simulink model "nms3D_2021"  (R2021a)
settings: Solver=ode15s  StartTime=0.0  StopTime=2  MaxStep=1e-2  RelTol=1e-2
StartFcn:
  | tic
StopFcn:
  | toc
  | 
  | 
  | %if GimbalLockFlag
  |  % fprintf(2, 'Almost reached Gimbal Lock of IMU. Simulation stopped.\n')
  | %end
  | 
  | %fprintf('Elapsed time: %4.2f sec (%4.2f%% realtime)\n', a, tout(end)/a*100)
values from neighbouring files (symbols this model uses):
  Balance02 = pMod(24:29)    [AssignSimulinkParams.m]    (also in assign_parameters.m = param(26:29))
  Balance13 = pMod(30:35)    [AssignSimulinkParams.m]    (also in assign_parameters.m = param(30:33))
  BalanceTrunk = pMod(22:23)    [AssignSimulinkParams.m]    (also in assign_parameters.m = param(22:23))
  BalanceTrunkLat = param(24:25)    [assign_parameters.m]
  BalanceTrunkLatOld = pMod(43:46)    [AssignSimulinkParams.m]    (also in assign_parameters.m = param(43:46))
  BalanceTrunkOld = param(49:53)    [assign_parameters.m]
  BasisStim = pMod(1:11)    [AssignSimulinkParams.m]    (also in assign_parameters.m = param(1:11))
  CompliantLeg = pMod(12:14)    [AssignSimulinkParams.m]    (also in assign_parameters.m = param(12:14))
  CompliantLegLat = pMod(15)    [AssignSimulinkParams.m]    (also in assign_parameters.m = param(15))
  PreventKneeOverextension = pMod(16:21)    [AssignSimulinkParams.m]    (also in assign_parameters.m = param(16:21))
  SwingCompLatOld = param(47:48)    [assign_parameters.m]
  Target02 = pMod(36:38)    [AssignSimulinkParams.m]    (also in assign_parameters.m = param(34:36))
  Target02_va = pMod(49:54)    [AssignSimulinkParams.m]    (also in assign_parameters.m = param(60:65))
  Target13 = pMod(39:41)    [AssignSimulinkParams.m]    (also in assign_parameters.m = param(37:39))
  Target13_va = pMod(55:60)    [AssignSimulinkParams.m]    (also in assign_parameters.m = param(66:71))
  theta0_world = param(59)    [assign_parameters.m]
  WramameiSL_1000 = readmatrix('WSL_1000_Norm_Sigmoid_MSE_cont.csv')    [nms3D_prep.m]
  ZramameiSL_1000 = readmatrix('ZSL_1000_Norm_Sigmoid_MSE_cont.csv')    [nms3D_prep.m]
undefined symbols (not defined in the file or in its folder): ICs, mParams, X, Y, Z
libraries: nesl_utility x106, sm_lib x87, simulink x70, eeGeneralControl x28, robotmaniplib x14, dspinverses x10, robotcorelib x5, dspmathops x3, vrlib x1, pid_lib x1
(part 3 of 8)

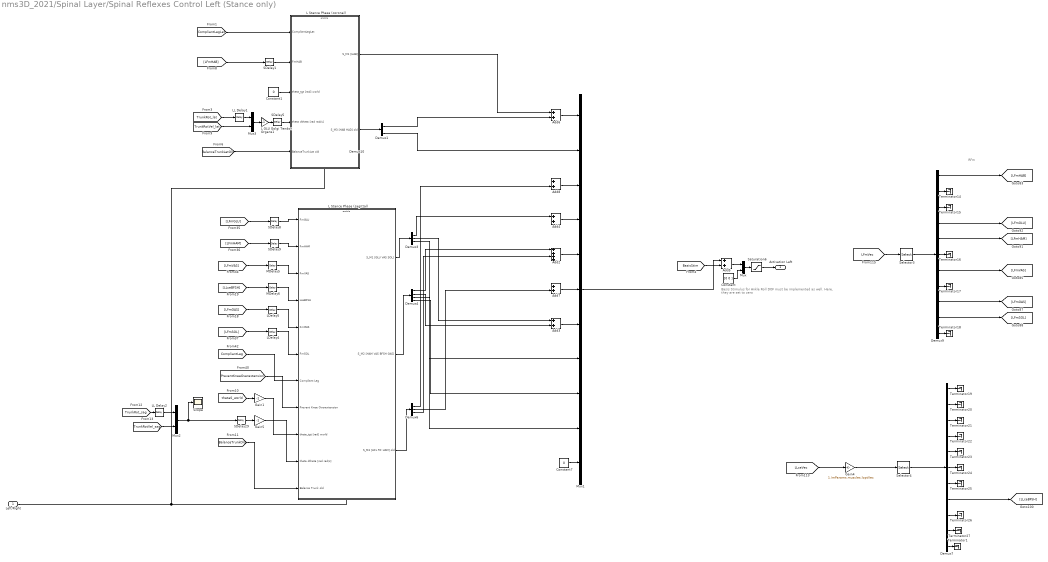
== system nms3D_2021/Spinal Layer/Spinal Reflexes Control Left (Stance only) ==
  note: Basis Stimulus for Ankle Roll DOF must be implemented as well.
      | Here, they are set to zero
  note: RFm
  Left/Right : Inport
  Add2 : Sum  Inputs=++++
  Add{3..8} (6 alike) : Sum
  Constant : Constant  Value=[0 0 ]
  Constant1 : Constant  Value=0
  Constant7 : Constant  Value=0
  Demux1 : Demux  Outputs=2
  Demux10 : Demux  Outputs=2
  Demux3 : Demux  Outputs=3
  Demux4 : Demux
  Demux6 : Demux  Outputs=3
  Demux7 : Demux  Outputs=11
  Demux9 : Demux  Outputs=11
  Gain1 : Gain  Gain=-1
  Gain4 : Gain  Gain=1./mParams.muscles.loptVec
  Gain5 : Gain  Gain=-1
  L GLU Golgi Tendon Organs1 : Gain  Gain=-1
  L Stance Phase (coronal) : Subsystem  TreatAsAtomicUnit=on
  L Stance Phase (sagittal) : Subsystem  TreatAsAtomicUnit=on
  LDelay4 : TransportDelay  DelayTime=mParams.control.delays.long
  LDelay5 : TransportDelay  DelayTime=mParams.control.delays.long
  LL Delay1 : TransportDelay  DelayTime=mParams.control.delays.longloop/2
  LL Delay2 : TransportDelay  DelayTime=mParams.control.delays.longloop/2
  MDelay5 : TransportDelay  DelayTime=mParams.control.delays.mid
  MDelay6 : TransportDelay  DelayTime=mParams.control.delays.mid
  Mux : Mux  Inputs=2
  Mux1 : Mux  Inputs=11
  Mux2 : Mux  Inputs=2
  Mux3 : Mux  Inputs=2
  SDelay{1,5,8..9,29} (5 alike) : TransportDelay  DelayTime=mParams.control.delays.short
  Saturation6 : Saturate  UpperLimit=1  LowerLimit=0.01  ZeroCross=off
  Scope : Scope
  Selector3 : Selector  InputPortWidth=13  IndexOptions=Index vector (dialog)  Indices=[1:11]  OutputSizes=1
  Selector4 : Selector  InputPortWidth=13  IndexOptions=Index vector (dialog)  Indices=[1:11]  OutputSizes=1
  Terminator{1,14..27} (15 alike) : Terminator
  Activation Left : Outport
  wires:
  [LFmVec] -> Selector3/1
  Demux9/1 -> [LFmHAB]
  Gain4/1 -> Selector4/1
  Demux9/5 -> [LFmHAM]
  Demux7/8 -> [LLceBFSH]
  Demux9/9 -> [LFmGAS]
  Demux9/10 -> [LFmSOL]
  Demux9/4 -> [LFmGLU]
  Demux9/7 -> [LFmVAS]
  Demux7/11 -> Terminator1/1
  Saturation6/1 -> Activation Left/1
  Left/Right/1 -> L Stance Phase (sagittal)/Enable, L Stance Phase (coronal)/Enable
  Demux9/2 -> Terminator14/1
  Demux9/3 -> Terminator15/1
  Demux9/6 -> Terminator16/1
  Demux9/8 -> Terminator17/1
  Demux9/11 -> Terminator18/1
  Demux7/1 -> Terminator19/1
  Demux7/2 -> Terminator20/1
  Demux7/3 -> Terminator21/1
  Demux7/4 -> Terminator22/1
  Demux7/5 -> Terminator23/1
  Demux7/6 -> Terminator24/1
  Demux7/7 -> Terminator25/1
  Demux7/9 -> Terminator26/1
  Demux7/10 -> Terminator27/1
  [BasisStim] -> Add5/2
  Mux1/1 -> Add5/1
  Constant7/1 -> Mux1/11
  Add2/1 -> Mux1/5
  Add3/1 -> Mux1/7
  [LFmGLU] -> SDelay8/1
  SDelay9/1 -> L Stance Phase (sagittal)/2(FmHAM)
  MDelay6/1 -> L Stance Phase (sagittal)/4(LceBFSH)
  [LLceBFSH] -> MDelay6/1
  [LFmSOL] -> LDelay4/1
  MDelay5/1 -> L Stance Phase (sagittal)/3(FmVAS)
  [LFmGAS] -> LDelay5/1
  LDelay5/1 -> L Stance Phase (sagittal)/5(FmGAS)
  SDelay8/1 -> L Stance Phase (sagittal)/1(FmGLU)
  [LFmHAM] -> SDelay9/1
  LDelay4/1 -> L Stance Phase (sagittal)/6(FmSOL)
  [LFmVAS] -> MDelay5/1
  [CompliantLeg] -> L Stance Phase (sagittal)/7(Compliant Leg)
  [PreventKneeOverextension] -> L Stance Phase (sagittal)/8(Prevent Knee Overextension)
  [CompliantLegLat] -> L Stance Phase (coronal)/1(CompliantLegLat)
  [LFmHAB] -> SDelay1/1
  Constant1/1 -> L Stance Phase (coronal)/3(theta_tgt [rad] world)
  SDelay1/1 -> L Stance Phase (coronal)/2(FmHAB)
  Add6/1 -> Mux1/1
  SDelay5/1 -> L Stance Phase (coronal)/4(theta dtheta [rad rad/s])
  [TrunkRotVel_lat] -> Mux3/2
  [TrunkRot_lat] -> LL Delay1/1
  LL Delay1/1 -> Mux3/1
  [BalanceTrunkLatOld] -> L Stance Phase (coronal)/5(BalanceTrunkLat old)
  [theta0_world] -> Gain1/1
  Gain1/1 -> L Stance Phase (sagittal)/9(theta_tgt [rad] world)
  Mux2/1 -> Scope/1, SDelay29/1
  SDelay29/1 -> Gain5/1
  LL Delay2/1 -> Mux2/1
  Gain5/1 -> L Stance Phase (sagittal)/10(theta dtheta [rad rad/s])
  [TrunkRot_sag] -> LL Delay2/1
  [TrunkRotVel_sag] -> Mux2/2
  [BalanceTrunkOld] -> L Stance Phase (sagittal)/11(Balance Trunk old)
  Mux3/1 -> L GLU Golgi Tendon Organs1/1
  L GLU Golgi Tendon Organs1/1 -> SDelay5/1
  L Stance Phase (coronal)/1(S_M1 [HAB]) -> Add6/1
  L Stance Phase (coronal)/2(S_M3 [HAB HAD] old) -> Demux1/1
  Demux1/1 -> Add6/2
  Demux1/2 -> Mux1/2
  L Stance Phase (sagittal)/1(S_M1 [GLU VAS SOL]) -> Demux3/1
  L Stance Phase (sagittal)/2(S_M2 [HAM VAS BFSH GAS]) -> Demux4/1
  L Stance Phase (sagittal)/3(S_M3 [HFL RF HAM] old) -> Demux6/1
  Add4/1 -> Mux1/4
  Demux3/1 -> Add4/1
  Demux4/1 -> Add2/1
  Demux6/3 -> Add2/3
  Add7/1 -> Mux1/6
  Add8/1 -> Mux1/3
  Demux6/1 -> Add8/2
  Demux6/2 -> Add7/2
  Demux3/2 -> Add3/1
  Demux4/2 -> Add3/2
  Demux4/3 -> Mux1/8
  Demux4/4 -> Mux1/9
  Demux3/3 -> Mux1/10
  Constant/1 -> Mux/2
  Add5/1 -> Mux/1
  Mux/1 -> Saturation6/1
  Selector3/1 -> Demux9/1
  [LLceVec] -> Gain4/1
  Selector4/1 -> Demux7/1

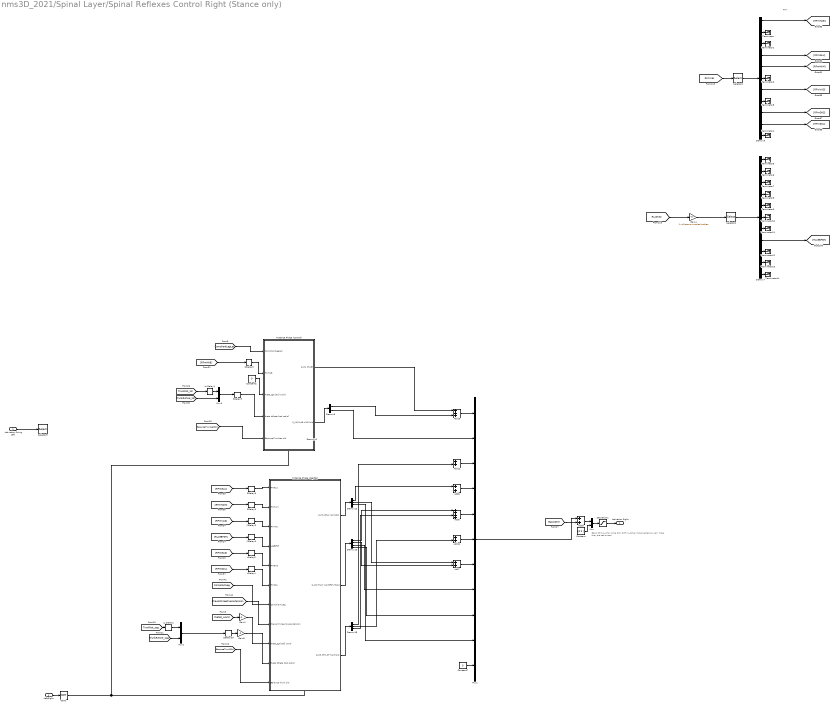
== system nms3D_2021/Spinal Layer/Spinal Reflexes Control Right (Stance only) ==
  note: RFm
  note: Basis Stimulus for Ankle Roll DOF must be implemented as well.
      | Here, they are set to zero
  Left/Right : Inport
  Activation Swing Left : Inport  Port=2
  Add10 : Sum  Inputs=+++
  Add{7..9,11..12} (5 alike) : Sum
  Add6 : Sum  Inputs=++++
  Constant : Constant  Value=[0 0 ]
  Constant1 : Constant  Value=0
  Constant7 : Constant  Value=0
  Demux10 : Demux  Outputs=2
  Demux12 : Demux  Outputs=3
  Demux13 : Demux
  Demux15 : Demux  Outputs=3
  Demux7 : Demux  Outputs=11
  Demux8 : Demux  Outputs=2
  Demux9 : Demux  Outputs=11
  Gain1 : Gain  Gain=-1
  Gain4 : Gain  Gain=1./mParams.muscles.loptVec
  Gain5 : Gain  Gain=-1
  LDelay4 : TransportDelay  DelayTime=mParams.control.delays.long
  LDelay5 : TransportDelay  DelayTime=mParams.control.delays.long
  LL Delay1 : TransportDelay  DelayTime=mParams.control.delays.longloop/2
  LL Delay2 : TransportDelay  DelayTime=mParams.control.delays.longloop/2
  MDelay5 : TransportDelay  DelayTime=mParams.control.delays.mid
  MDelay6 : TransportDelay  DelayTime=mParams.control.delays.mid
  Mux : Mux  Inputs=2
  Mux1 : Mux  Inputs=11
  Mux2 : Mux  Inputs=2
  Mux3 : Mux  Inputs=2
  NOT1 : Logic  Operator=NOT  AllPortsSameDT=off  OutDataTypeStr=boolean
  R Stance Phase (coronal) : Subsystem  TreatAsAtomicUnit=on
  R Stance Phase (sagittal) : Subsystem  TreatAsAtomicUnit=on
  SDelay{3,5,8..9,29} (5 alike) : TransportDelay  DelayTime=mParams.control.delays.short
  Saturation1 : Saturate  UpperLimit=1  LowerLimit=0.01  ZeroCross=off
  Selector1 : Selector  InputPortWidth=13  IndexOptions=Index vector (dialog)  Indices=[1:11]  OutputSizes=1
  Selector2 : Selector  InputPortWidth=13  IndexOptions=Index vector (dialog)  Indices=[1:11]  OutputSizes=1
  Selector5 : Selector  InputPortWidth=13  IndexOptions=Index vector (dialog)  Indices=[1:11]  OutputSizes=1
  Terminator{,1..14} (15 alike) : Terminator
  Activation Right : Outport
  wires:
  [RFmVec] -> Selector1/1
  Demux9/1 -> [RFmHAB]
  Gain4/1 -> Selector2/1
  Demux9/5 -> [RFmHAM]
  Demux7/8 -> [RLceBFSH]
  Demux9/9 -> [RFmGAS]
  Demux9/10 -> [RFmSOL]
  Demux9/4 -> [RFmGLU]
  Demux9/7 -> [RFmVAS]
  Demux7/11 -> Terminator14/1
  Demux9/2 -> Terminator/1
  Demux9/3 -> Terminator1/1
  Demux9/6 -> Terminator2/1
  Demux9/8 -> Terminator3/1
  Demux9/11 -> Terminator4/1
  Demux7/1 -> Terminator5/1
  Demux7/2 -> Terminator6/1
  Demux7/3 -> Terminator7/1
  Demux7/4 -> Terminator8/1
  Demux7/5 -> Terminator9/1
  Demux7/6 -> Terminator10/1
  Demux7/7 -> Terminator11/1
  Demux7/9 -> Terminator12/1
  Demux7/10 -> Terminator13/1
  [RFmHAB] -> SDelay3/1
  LL Delay1/1 -> Mux3/1
  [CompliantLeg] -> R Stance Phase (sagittal)/7(Compliant Leg)
  [theta0_world] -> Gain1/1
  Demux13/1 -> Add6/1
  Left/Right/1 -> NOT1/1
  Gain1/1 -> R Stance Phase (sagittal)/9(theta_tgt [rad] world)
  Demux12/2 -> Add7/1
  [RFmGLU] -> SDelay8/1
  SDelay8/1 -> R Stance Phase (sagittal)/1(FmGLU)
  [RLceBFSH] -> MDelay6/1
  Add6/1 -> Mux1/5
  Demux12/3 -> Mux1/10
  MDelay6/1 -> R Stance Phase (sagittal)/4(LceBFSH)
  Mux3/1 -> SDelay5/1
  R Stance Phase (sagittal)/3(S_M3 [HFL RF HAM] old) -> Demux15/1
  Demux13/4 -> Mux1/9
  [RFmGAS] -> LDelay5/1
  Constant7/1 -> Mux1/11
  [RFmSOL] -> LDelay4/1
  SDelay9/1 -> R Stance Phase (sagittal)/2(FmHAM)
  [TrunkRot_lat] -> LL Delay1/1
  LDelay4/1 -> R Stance Phase (sagittal)/6(FmSOL)
  [BasisStim] -> Add9/2
  Add10/1 -> Mux1/1
  Add7/1 -> Mux1/7
  Mux1/1 -> Add9/1
  Add12/1 -> Mux1/3
  Saturation1/1 -> Activation Right/1
  R Stance Phase (coronal)/1(S_M1 [HAB]) -> Add10/1
  Demux15/2 -> Add11/2
  [RFmVAS] -> MDelay5/1
  Demux13/2 -> Add7/2
  Demux13/3 -> Mux1/8
  R Stance Phase (coronal)/2(S_M3 [HAB HAD] old) -> Demux8/1
  Add11/1 -> Mux1/6
  Demux8/2 -> Mux1/2
  Demux15/3 -> Add6/3
  [RFmHAM] -> SDelay9/1
  Add8/1 -> Mux1/4
  SDelay5/1 -> R Stance Phase (coronal)/4(theta dtheta [rad rad/s])
  Demux15/1 -> Add12/2
  Demux12/1 -> Add8/1
  Activation Swing Left/1 -> Selector5/1
  R Stance Phase (sagittal)/2(S_M2 [HAM VAS BFSH GAS]) -> Demux13/1
  R Stance Phase (sagittal)/1(S_M1 [GLU VAS SOL]) -> Demux12/1
  Gain5/1 -> R Stance Phase (sagittal)/10(theta dtheta [rad rad/s])
  [BalanceTrunkOld] -> R Stance Phase (sagittal)/11(Balance Trunk old)
  Demux8/1 -> Add10/3
  LDelay5/1 -> R Stance Phase (sagittal)/5(FmGAS)
  [PreventKneeOverextension] -> R Stance Phase (sagittal)/8(Prevent Knee Overextension)
  [TrunkRotVel_sag] -> Mux2/2
  MDelay5/1 -> R Stance Phase (sagittal)/3(FmVAS)
  [TrunkRot_sag] -> LL Delay2/1
  [TrunkRotVel_lat] -> Mux3/2
  Mux2/1 -> SDelay29/1
  [BalanceTrunkLatOld] -> R Stance Phase (coronal)/5(BalanceTrunkLat old)
  [CompliantLegLat] -> R Stance Phase (coronal)/1(CompliantLegLat)
  LL Delay2/1 -> Mux2/1
  SDelay29/1 -> Gain5/1
  SDelay3/1 -> R Stance Phase (coronal)/2(FmHAB)
  Constant1/1 -> R Stance Phase (coronal)/3(theta_tgt [rad] world)
  NOT1/1 -> R Stance Phase (sagittal)/Enable, R Stance Phase (coronal)/Enable
  Constant/1 -> Mux/2
  Mux/1 -> Saturation1/1
  Add9/1 -> Mux/1
  Selector1/1 -> Demux9/1
  [RLceVec] -> Gain4/1
  Selector2/1 -> Demux7/1

== system nms3D_2021/Spinal Layer/Stretch Reflex ==
  Descending Commands Left : Inport
  Descending Commands Right : Inport  Port=2
  Filtered Derivative (Discrete or Continuous)1 : eeGeneralControl/Filtered Derivative (Discrete or Continuous)  K=1  T=0.0025  B=inf  A=-inf  minRatio=10  init_option=Inherited from block input  x0=0  Ts=0
      settings: SourceProductBaseCode=PS
  Filtered Derivative (Discrete or Continuous)2 : eeGeneralControl/Filtered Derivative (Discrete or Continuous)  K=1  T=0.0025  B=inf  A=-inf  minRatio=10  init_option=Inherited from block input  x0=0  Ts=0
      settings: SourceProductBaseCode=PS
  Saturation1 : Saturate  UpperLimit=1  LowerLimit=0  ZeroCross=off
  Saturation4 : Saturate  UpperLimit=1  LowerLimit=0  ZeroCross=off
  Stretch Reflex Left : Subsystem
  Stretch Reflex Right : Subsystem
  Time Delay{,1..5} (6 alike) : eeGeneralControl/Low-Pass Filter (Discrete or Continuous)  K=1  T=0.0025  B=inf  A=-inf  init_option=Inherited from block input  x0=0  Ts=0
  Activation Left : Outport
  Activation Right : Outport  Port=2
  wires:
  Descending Commands Left/1 -> Time Delay/1, Filtered Derivative (Discrete or Continuous)2/1
  Filtered Derivative (Discrete or Continuous)1/1 -> Stretch Reflex Right/4(lambda_dot)
  Descending Commands Right/1 -> Time Delay3/1, Filtered Derivative (Discrete or Continuous)1/1
  Stretch Reflex Right/1(STIM) -> Saturation4/1
  Stretch Reflex Left/1(STIM) -> Saturation1/1
  Filtered Derivative (Discrete or Continuous)2/1 -> Stretch Reflex Left/4(lambda_dot)
  [LLceVec] -> Time Delay1/1
  [LVceVec] -> Time Delay2/1
  [RVceVec] -> Time Delay5/1
  [RLceVec] -> Time Delay4/1
  Time Delay2/1 -> Stretch Reflex Left/3(v_ce)
  Time Delay1/1 -> Stretch Reflex Left/2(l_ce)
  Time Delay/1 -> Stretch Reflex Left/1(lambda)
  Time Delay4/1 -> Stretch Reflex Right/2(l_ce)
  Time Delay5/1 -> Stretch Reflex Right/3(v_ce)
  Time Delay3/1 -> Stretch Reflex Right/1(lambda)
  Saturation1/1 -> Activation Left/1
  Saturation4/1 -> Activation Right/1

== system nms3D_2021/Supraspinal Level/Finite State Machine ==
  note: Finite State Machine (FSM): The FSM comprises 4 states (Early Right Swing (0), Late Right Swing (1), Early Left Swing (2) and Late Left Swing (3)). The FSM transitions from state 0 to state 1 and from state 2 to state 3 when the time dt in state 0/2 is passed. It transitions from state 2 to state 3 and from state 3 to state 1 when right/left contact is measured.
  Information: Ground Contact : Inport
  Chart : Stateflow chart  TreatAsAtomicUnit=on
  Constant : Constant  Value=0.3
  Demux : Demux  Outputs=2
  Early Right Swing : Outport
  Late Right Swing : Outport  Port=2
  Early Left Swing : Outport  Port=3
  Late Left Swing : Outport  Port=4
  wires:
  Demux/1 -> Chart/2(contact_left)
  Constant/1 -> Chart/1(dt)
  Demux/2 -> Chart/3(contact_right)
  Information: Ground Contact/1 -> Demux/1
  Chart/1(state0) -> Early Right Swing/1
  Chart/2(state1) -> Late Right Swing/1
  Chart/3(state2) -> Early Left Swing/1
  Chart/4(state3) -> Late Left Swing/1

== system nms3D_2021/Supraspinal Level/Subsystem ==
  note: Force Inversion
  note: Muscle Inversion
  note: Stretch Reflex Inversion
  note: The interaction wrench contains the wrench that the swing leg motion applies to the stance leg. This might be used for interaction compensation
  Early/Late Swing : Inport
  Swing Right : Inport  Port=2
  Compute positives forces that generate desired torque profiles1 : Subsystem
  Inversion of Muscle Model : Subsystem
  NOT : Logic  Operator=NOT  AllPortsSameDT=off  OutDataTypeStr=boolean
  Product2 : Product
  Product3 : Product
  Stance Leg Control : Subsystem
  Stretch Reflex Inversion : Subsystem
  Swing Leg Control : Subsystem
  Terminator : Terminator
  Terminator1 : Terminator
  Descending Command Left : Outport
  Descending Command Right : Outport  Port=2
  wires:
  Stretch Reflex Inversion/2(Descending Command Right) -> Descending Command Right/1
  Inversion of Muscle Model/1(Desired Activation Left) -> Stretch Reflex Inversion/1(Desired Activation Left)
  Stretch Reflex Inversion/1(Descending Command Left) -> Descending Command Left/1
  Inversion of Muscle Model/2(Desired Activation Right) -> Stretch Reflex Inversion/2(Desired Activation Right)
  Early/Late Swing/1 -> Swing Leg Control/2(Early/Late Swing)
  Swing Leg Control/1(Desired Torques Left Swing) -> Compute positives forces that generate desired torque profiles1/3(Swing Left)
  Swing Leg Control/2(Desired Torques Right Swing) -> Compute positives forces that generate desired torque profiles1/4(Swing Right)
  Stance Leg Control/1(Push Off Left) -> Product2/1
  Stance Leg Control/2(Push Off Right) -> Product3/1
  Product2/1 -> Compute positives forces that generate desired torque profiles1/2(Stance Left)
  Swing Right/1 -> Compute positives forces that generate desired torque profiles1/1(Left/Right), NOT/1, Product2/2, Stance Leg Control/1(Left/Right), Swing Leg Control/1(Left/Right)
  Product3/1 -> Compute positives forces that generate desired torque profiles1/5(Stance Right)
  NOT/1 -> Product3/2
  Compute positives forces that generate desired torque profiles1/1(Desired Force) -> Inversion of Muscle Model/1(Desired Forces)
  Swing Leg Control/3(Interaction Wrench Right) -> Terminator/1
  Swing Leg Control/4(Interaction Wrench Left) -> Terminator1/1

== system nms3D_2021/Body and Contact Model/L Leg/Ankle Mechanical Limits ==
  note: Overextension Torque
  note: Joint Limits
  note: Overflexion Torque
  dq [rad/s] : Inport
  q [rad] : Inport  Port=2
  Gain1 : Gain  Gain=mParams.joints.ankle.kStop
  Gain2 : Gain  Gain=-1
  Gain3 : Gain  Gain=mParams.joints.ankle.kStop
  Gain4 : Gain  Gain=1/mParams.joints.ankle.wMaxStop
  Gain5 : Gain  Gain=-1
  Gain6 : Gain  Gain=-1
  Limit Knee Range : simulink/Logic and Bit Operations/Interval Test  IntervalClosedRight=on  uplimit=mParams.joints.ankle.MaxPitch + 20*pi/180  IntervalClosedLeft=on  lowlimit=mParams.joints.ankle.MinPitch - 20*pi/180  OutDataTypeStr=boolean
      settings: AttributesFormatString=|
      | Lower limits: %<lowlimit>
      | Upper limits: %<uplimit>
  Logical Operator3 : Logic  Operator=NOT  AllPortsSameDT=off  OutDataTypeStr=boolean
  Product1 : Product  Inputs=4
  Product2 : Product  Inputs=4
  Stop Simulation1 : Stop
  Sum : Sum  Inputs=|+-
  Sum1 : Sum  Inputs=|+-
  Sum2 : Sum
  Sum3 : Sum  Inputs=|-+
  Sum4 : Sum  Inputs=|-+
  above upper limit? : simulink/Logic and Bit Operations/Compare To Zero  relop=>  OutDataTypeStr=boolean  ZeroCross=off
  below lower limit? : simulink/Logic and Bit Operations/Compare To Zero  relop=<  OutDataTypeStr=boolean  ZeroCross=off
  const : Constant
  const1 : Constant
  mech limit pushes back? : simulink/Logic and Bit Operations/Compare To Zero  relop=>  OutDataTypeStr=boolean  ZeroCross=off
  mech limit pushes back?. : simulink/Logic and Bit Operations/Compare To Zero  relop=>  OutDataTypeStr=boolean  ZeroCross=off
  overextension angle : Constant  Value=mParams.joints.ankle.MaxPitch
  overflexion angle : Constant  Value=mParams.joints.ankle.MinPitch
  tau [Nm] : Outport  VectorParamsAs1DForOutWhenUnconnected=off
  wires:
  Logical Operator3/1 -> Stop Simulation1/1
  Limit Knee Range/1 -> Logical Operator3/1
  Gain6/1 -> Sum2/1
  Gain2/1 -> Sum3/1
  Sum2/1 -> tau [Nm]/1
  overflexion angle/1 -> Sum1/2
  Sum1/1 -> Gain1/1
  Sum/1 -> Gain3/1
  q [rad]/1 -> Sum1/1, Limit Knee Range/1, Sum/1
  overextension angle/1 -> Sum/2
  dq [rad/s]/1 -> Gain4/1
  const/1 -> Sum3/2
  Sum3/1 -> Product1/3, mech limit pushes back?/1
  Gain3/1 -> Product1/2, above upper limit?/1
  mech limit pushes back?/1 -> Product1/4
  above upper limit?/1 -> Product1/1
  Product1/1 -> Gain6/1
  Product2/1 -> Gain5/1
  below lower limit?/1 -> Product2/1
  mech limit pushes back?./1 -> Product2/4
  Gain1/1 -> below lower limit?/1, Product2/2
  Sum4/1 -> mech limit pushes back?./1, Product2/3
  const1/1 -> Sum4/2
  Gain4/1 -> Sum4/1, Gain2/1
  Gain5/1 -> Sum2/2

== system nms3D_2021/Body and Contact Model/L Leg/Foot ==
  "  XYZ Sensor Ball left1" : Subsystem
  B Transform : sm_lib/Frames and Transforms/Rigid Transform  TranslationMethod=Cartesian  TranslationStandardOffset=0  TranslationLengthUnit=m  TranslationStandardAxis=+Y  TranslationCartesianOffset=[ mParams.bodies.foot.compensation mParams.bodies.foot.l/2 0]  TranslationROffset=0  TranslationROffsetUnits=m  TranslationZOffset=0  TranslationZOffsetUnits=m  TranslationThetaOffset=0  TranslationThetaOffsetUnits=deg  RotationMethod=None  RotationAngleUnits=deg  RotationStandardAxis=+X  RotationAngle=90  RotationArbitraryAxis=[0 0 1]  FollAlignAxisA=+X  BaseAlignAxisA=+Y  FollAlignAxisB=+Y  BaseAlignAxisB=+Z  RotationSequenceAxes=FollowerAxes  RotationSequence=XYX  RotationSequenceAngles=[0 0 0]  RotationSequenceAnglesUnits=deg  RotationMatrix=[1 0 0; 0 1 0; 0 0 1]
  LB Transform : sm_lib/Frames and Transforms/Rigid Transform  TranslationMethod=Cartesian  TranslationStandardOffset=0  TranslationLengthUnit=m  TranslationStandardAxis=+Y  TranslationCartesianOffset="[mParams.bodies.foot.l/2 -mParams.bodies.foot.compensation  -mParams.bodies.foot.BallWidth/2]"  TranslationROffset=0  TranslationROffsetUnits=m  TranslationZOffset=0  TranslationZOffsetUnits=m  TranslationThetaOffset=0  TranslationThetaOffsetUnits=deg  RotationMethod=None  RotationAngleUnits=deg  RotationStandardAxis=+X  RotationAngle=90  RotationArbitraryAxis=[0 0 1]  FollAlignAxisA=+X  BaseAlignAxisA=+Y  FollAlignAxisB=+Y  BaseAlignAxisB=+Z  RotationSequenceAxes=FollowerAxes  RotationSequence=XYX  RotationSequenceAngles=[0 0 0]  RotationSequenceAnglesUnits=deg  RotationMatrix=[1 0 0; 0 1 0; 0 0 1]
  LH Transform : sm_lib/Frames and Transforms/Rigid Transform  TranslationMethod=Cartesian  TranslationStandardOffset=0  TranslationLengthUnit=m  TranslationStandardAxis=+Y  TranslationCartesianOffset="[-mParams.bodies.foot.l/2 -mParams.bodies.foot.compensation  -mParams.bodies.foot.HeelWidth/2]"  TranslationROffset=0  TranslationROffsetUnits=m  TranslationZOffset=0  TranslationZOffsetUnits=m  TranslationThetaOffset=0  TranslationThetaOffsetUnits=deg  RotationMethod=None  RotationAngleUnits=deg  RotationStandardAxis=+X  RotationAngle=90  RotationArbitraryAxis=[0 0 1]  FollAlignAxisA=+X  BaseAlignAxisA=+Y  FollAlignAxisB=+Y  BaseAlignAxisB=+Z  RotationSequenceAxes=FollowerAxes  RotationSequence=XYX  RotationSequenceAngles=[0 0 0]  RotationSequenceAnglesUnits=deg  RotationMatrix=[1 0 0; 0 1 0; 0 0 1]
  RB Transform : sm_lib/Frames and Transforms/Rigid Transform  TranslationMethod=Cartesian  TranslationStandardOffset=0  TranslationLengthUnit=m  TranslationStandardAxis=+Z  TranslationCartesianOffset="[mParams.bodies.foot.l/2 -mParams.bodies.foot.compensation  mParams.bodies.foot.BallWidth/2]"  TranslationROffset=0  TranslationROffsetUnits=m  TranslationZOffset=0  TranslationZOffsetUnits=m  TranslationThetaOffset=0  TranslationThetaOffsetUnits=deg  RotationMethod=None  RotationAngleUnits=deg  RotationStandardAxis=+Z  RotationAngle=0.0  RotationArbitraryAxis=[0 0 1]  FollAlignAxisA=+X  BaseAlignAxisA=+Y  FollAlignAxisB=+Y  BaseAlignAxisB=+Z  RotationSequenceAxes=FollowerAxes  RotationSequence=XYX  RotationSequenceAngles=[0 0 0]  RotationSequenceAnglesUnits=deg  RotationMatrix=[1 0 0; 0 1 0; 0 0 1]
  RH Transform : sm_lib/Frames and Transforms/Rigid Transform  TranslationMethod=Cartesian  TranslationStandardOffset=0  TranslationLengthUnit=m  TranslationStandardAxis=+Z  TranslationCartesianOffset="[-mParams.bodies.foot.l/2 -mParams.bodies.foot.compensation  mParams.bodies.foot.HeelWidth/2]"  TranslationROffset=0  TranslationROffsetUnits=m  TranslationZOffset=0  TranslationZOffsetUnits=m  TranslationThetaOffset=0  TranslationThetaOffsetUnits=deg  RotationMethod=None  RotationAngleUnits=deg  RotationStandardAxis=+Z  RotationAngle=0.0  RotationArbitraryAxis=[0 0 1]  FollAlignAxisA=+X  BaseAlignAxisA=+Y  FollAlignAxisB=+Y  BaseAlignAxisB=+Z  RotationSequenceAxes=FollowerAxes  RotationSequence=XYX  RotationSequenceAngles=[0 0 0]  RotationSequenceAnglesUnits=deg  RotationMatrix=[1 0 0; 0 1 0; 0 0 1]
  Solid1 : sm_lib/Body Elements/Brick Solid  GraphicAmbientColor=[0.15 0.15 0.15 1.0]  BasedOnType=Density  BrickDimensions="[mParams.bodies.foot.l  mParams.bodies.foot.d mParams.bodies.foot.b]"  BrickDimensionUnits=m  CenterOfMass=mParams.bodies.foot.CG  CenterOfMassUnits=m  GraphicDiffuseColor=[1 0.5 0.5]  Density=2.7  DensityUnits=g/cm^3  DoExposeReferenceFrame=on  GraphicEmissiveColor=[0 0 0 1.0]  ExportEntireGeometry=off  SerializedFrames=<Frames><Frame><Id>Frame1</Id><Value><Name>CG</Name><Origin><Source>CenterOfMassFrame</Source><FeatureName></FeatureName></Origin><PrimaryAxis><DefinedDirection>+Z</DefinedDirection><Source>ReferenceFrame</Source><SourceDirection>+Z</SourceDirection><FeatureName></FeatureName></PrimaryAxis><SecondaryAxis><DefinedDirection>+X</DefinedDirection><Source>ReferenceFrame</Source><SourceDirection>+X</SourceDirection><FeatureName></FeatureName></SecondaryAxis></Value></Frame></Frames>  MarkerShape=Sphere  MarkerSize=10  GraphicType=FromGeometry  InertiaType=Custom  Mass=mParams.bodies.foot.m  MassUnits=kg  MomentsOfInertia=mParams.bodies.foot.In  MomentsOfInertiaUnits=kg*m^2  GraphicOpacity=1.0  ProductsOfInertia=[0 0 0]  ProductsOfInertiaUnits=kg*m^2  GraphicShininess=75  GraphicSpecularColor=[0.5 0.5 0.5 1.0]  GraphicVisPropType=SimpleVisualProperties
  Terminator2 : Terminator
  Transform CS1(Ankle) to MidSegment1 : sm_lib/Frames and Transforms/Rigid Transform  TranslationMethod=Cartesian  TranslationStandardOffset=0  TranslationLengthUnit=m  TranslationStandardAxis=+Y  TranslationCartesianOffset=mParams.bodies.foot.AnkleToMid  TranslationROffset=0  TranslationROffsetUnits=m  TranslationZOffset=0  TranslationZOffsetUnits=m  TranslationThetaOffset=0  TranslationThetaOffsetUnits=deg  RotationMethod=RotationSequence  RotationAngleUnits=deg  RotationStandardAxis=+X  RotationAngle=-90  RotationArbitraryAxis=[0 0 1]  FollAlignAxisA=+X  BaseAlignAxisA=+Y  FollAlignAxisB=+Y  BaseAlignAxisB=+Z  RotationSequenceAxes=FollowerAxes  RotationSequence=ZXY  RotationSequenceAngles=[90 0 0]  RotationSequenceAnglesUnits=deg  RotationMatrix=[1 0 0; 0 1 0; 0 0 1]
  CS1 : PMIOPort  Side=Left
  Left Ball : PMIOPort  Port=2  Side=Right
  Left Heel : PMIOPort  Port=3  Side=Left
  Right Ball : PMIOPort  Port=4  Side=Right
  Right Heel : PMIOPort  Port=5  Side=Left
  tag scope: Ball_left=global, RotationMatrixLeftFoot=global
  wires:
  "  XYZ Sensor Ball left1"/2(v_bLH [m/s x3]) -> Terminator2/1
  "  XYZ Sensor Ball left1"/1(p_bLH [m x3]) -> [Ball_left]
  "  XYZ Sensor Ball left1"/3(Rotation Matrix) -> [RotationMatrixLeftFoot]
  connections:
  Transform CS1(Ankle) to MidSegment1/RConn1 -- Solid1/RConn1 -- RB Transform/LConn1 -- RH Transform/LConn1 -- B Transform/LConn1 -- LH Transform/LConn1 -- LB Transform/LConn1
  Transform CS1(Ankle) to MidSegment1/LConn1 -- CS1/RConn1
  Left Heel/RConn1 -- LH Transform/RConn1
  Left Ball/RConn1 -- LB Transform/RConn1
  Right Heel/RConn1 -- RH Transform/RConn1
  Right Ball/RConn1 -- RB Transform/RConn1
  B Transform/RConn1 -- "  XYZ Sensor Ball left1"/LConn1

== system nms3D_2021/Body and Contact Model/L Leg/Hip Pitch Mechanical Limits ==
  note: Overflexion Torque
  note: Joint Limits
  note: Overextension Torque
  dq [rad/s] : Inport
  q [rad] : Inport  Port=2
  Gain1 : Gain  Gain=mParams.joints.hip.kStop
  Gain2 : Gain  Gain=-1
  Gain3 : Gain  Gain=mParams.joints.hip.kStop
  Gain4 : Gain  Gain=1/mParams.joints.hip.wMaxStop
  Gain5 : Gain  Gain=-1
  Gain6 : Gain  Gain=-1
  Limit Joint Range : simulink/Logic and Bit Operations/Interval Test  IntervalClosedRight=on  uplimit=mParams.joints.hip.MaxPitch + 20*pi/180  IntervalClosedLeft=on  lowlimit=mParams.joints.hip.MinPitch - 20*pi/180  OutDataTypeStr=boolean
      settings: AttributesFormatString=|
      | Lower limits: %<lowlimit>
      | Upper limits: %<uplimit>
  Logical Operator3 : Logic  Operator=NOT  AllPortsSameDT=off  OutDataTypeStr=boolean
  Product1 : Product  Inputs=4
  Product2 : Product  Inputs=4
  Stop Simulation1 : Stop
  Sum : Sum  Inputs=|+-
  Sum1 : Sum  Inputs=|+-
  Sum2 : Sum
  Sum3 : Sum  Inputs=|-+
  Sum4 : Sum  Inputs=|-+
  above upper limit? : simulink/Logic and Bit Operations/Compare To Zero  relop=>  OutDataTypeStr=boolean  ZeroCross=off
  below lower limit? : simulink/Logic and Bit Operations/Compare To Zero  relop=<  OutDataTypeStr=boolean  ZeroCross=off
  const : Constant
  const1 : Constant
  mech limit pushes back? : simulink/Logic and Bit Operations/Compare To Zero  relop=>  OutDataTypeStr=boolean  ZeroCross=off
  mech limit pushes back?. : simulink/Logic and Bit Operations/Compare To Zero  relop=>  OutDataTypeStr=boolean  ZeroCross=off
  overextension angle : Constant  Value=mParams.joints.hip.MaxPitch
  overflexion angle : Constant  Value=mParams.joints.hip.MinPitch
  tau [Nm] : Outport  VectorParamsAs1DForOutWhenUnconnected=off
  wires:
  Gain5/1 -> Sum2/2
  Gain4/1 -> Gain2/1, Sum4/1
  const1/1 -> Sum4/2
  Sum4/1 -> Product2/3, mech limit pushes back?./1
  Gain1/1 -> below lower limit?/1, Product2/2
  mech limit pushes back?./1 -> Product2/4
  below lower limit?/1 -> Product2/1
  Product2/1 -> Gain5/1
  Product1/1 -> Gain6/1
  above upper limit?/1 -> Product1/1
  mech limit pushes back?/1 -> Product1/4
  Gain3/1 -> above upper limit?/1, Product1/2
  Sum3/1 -> mech limit pushes back?/1, Product1/3
  const/1 -> Sum3/2
  dq [rad/s]/1 -> Gain4/1
  overextension angle/1 -> Sum/2
  q [rad]/1 -> Limit Joint Range/1, Sum1/1, Sum/1
  Sum/1 -> Gain3/1
  Sum1/1 -> Gain1/1
  overflexion angle/1 -> Sum1/2
  Sum2/1 -> tau [Nm]/1
  Gain2/1 -> Sum3/1
  Gain6/1 -> Sum2/1
  Limit Joint Range/1 -> Logical Operator3/1
  Logical Operator3/1 -> Stop Simulation1/1

== system nms3D_2021/Body and Contact Model/L Leg/Hip Roll Mechanical Limits ==
  note: Overflexion Torque
  note: Joint Limits
  note: Overextension Torque
  dq [rad/s] : Inport
  q [rad] : Inport  Port=2
  Gain1 : Gain  Gain=mParams.joints.hip.kStop
  Gain2 : Gain  Gain=-1
  Gain3 : Gain  Gain=mParams.joints.hip.kStop
  Gain4 : Gain  Gain=1/mParams.joints.hip.wMaxStop
  Gain5 : Gain  Gain=-1
  Gain6 : Gain  Gain=-1
  Limit Joint Range : simulink/Logic and Bit Operations/Interval Test  IntervalClosedRight=on  uplimit=mParams.joints.hip.MaxRoll + 20*pi/180  IntervalClosedLeft=on  lowlimit=mParams.joints.hip.MinRoll - 20*pi/180  OutDataTypeStr=boolean
      settings: AttributesFormatString=|
      | Lower limits: %<lowlimit>
      | Upper limits: %<uplimit>
  Logical Operator3 : Logic  Operator=NOT  AllPortsSameDT=off  OutDataTypeStr=boolean
  Product1 : Product  Inputs=4
  Product2 : Product  Inputs=4
  Stop Simulation1 : Stop
  Sum : Sum  Inputs=|+-
  Sum1 : Sum  Inputs=|+-
  Sum2 : Sum
  Sum3 : Sum  Inputs=|-+
  Sum4 : Sum  Inputs=|-+
  above upper limit? : simulink/Logic and Bit Operations/Compare To Zero  relop=>  OutDataTypeStr=boolean  ZeroCross=off
  below lower limit? : simulink/Logic and Bit Operations/Compare To Zero  relop=<  OutDataTypeStr=boolean  ZeroCross=off
  const : Constant
  const1 : Constant
  mech limit pushes back? : simulink/Logic and Bit Operations/Compare To Zero  relop=>  OutDataTypeStr=boolean  ZeroCross=off
  mech limit pushes back?. : simulink/Logic and Bit Operations/Compare To Zero  relop=>  OutDataTypeStr=boolean  ZeroCross=off
  overextension angle : Constant  Value=mParams.joints.hip.MaxRoll
  overflexion angle : Constant  Value=mParams.joints.hip.MinRoll
  tau [Nm] : Outport  VectorParamsAs1DForOutWhenUnconnected=off
  wires:
  Gain5/1 -> Sum2/2
  Gain4/1 -> Gain2/1, Sum4/1
  const1/1 -> Sum4/2
  Sum4/1 -> Product2/3, mech limit pushes back?./1
  Gain1/1 -> below lower limit?/1, Product2/2
  mech limit pushes back?./1 -> Product2/4
  below lower limit?/1 -> Product2/1
  Product2/1 -> Gain5/1
  Product1/1 -> Gain6/1
  above upper limit?/1 -> Product1/1
  mech limit pushes back?/1 -> Product1/4
  Gain3/1 -> above upper limit?/1, Product1/2
  Sum3/1 -> mech limit pushes back?/1, Product1/3
  const/1 -> Sum3/2
  dq [rad/s]/1 -> Gain4/1
  overextension angle/1 -> Sum/2
  q [rad]/1 -> Limit Joint Range/1, Sum1/1, Sum/1
  Sum/1 -> Gain3/1
  Sum1/1 -> Gain1/1
  overflexion angle/1 -> Sum1/2
  Sum2/1 -> tau [Nm]/1
  Gain2/1 -> Sum3/1
  Gain6/1 -> Sum2/1
  Limit Joint Range/1 -> Logical Operator3/1
  Logical Operator3/1 -> Stop Simulation1/1

== system nms3D_2021/Body and Contact Model/L Leg/Knee Mechanical Limits ==
  note: Overflexion Torque
  note: Joint Limits
  note: Overextension Torque
  dq [rad/s] : Inport
  q [rad] : Inport  Port=2
  Gain1 : Gain  Gain=mParams.joints.knee.kStop
  Gain2 : Gain  Gain=-1
  Gain3 : Gain  Gain=mParams.joints.knee.kStop
  Gain4 : Gain  Gain=1/mParams.joints.knee.wMaxStop
  Gain5 : Gain  Gain=-1
  Gain6 : Gain  Gain=-1
  Limit Knee Range : simulink/Logic and Bit Operations/Interval Test  IntervalClosedRight=on  uplimit=mParams.joints.knee.MaxPitch + 20*pi/180  IntervalClosedLeft=on  lowlimit=mParams.joints.knee.MinPitch - 20*pi/180  OutDataTypeStr=boolean
      settings: AttributesFormatString=|
      | Lower limits: %<lowlimit>
      | Upper limits: %<uplimit>
  Logical Operator3 : Logic  Operator=NOT  AllPortsSameDT=off  OutDataTypeStr=boolean
  Product1 : Product  Inputs=4
  Product2 : Product  Inputs=4
  Stop Simulation1 : Stop
  Sum : Sum  Inputs=|+-
  Sum1 : Sum  Inputs=|+-
  Sum2 : Sum
  Sum3 : Sum  Inputs=|-+
  Sum4 : Sum  Inputs=|-+
  above upper limit? : simulink/Logic and Bit Operations/Compare To Zero  relop=>  OutDataTypeStr=boolean  ZeroCross=off
  below lower limit? : simulink/Logic and Bit Operations/Compare To Zero  relop=<  OutDataTypeStr=boolean  ZeroCross=off
  const : Constant
  const1 : Constant
  mech limit pushes back? : simulink/Logic and Bit Operations/Compare To Zero  relop=>  OutDataTypeStr=boolean  ZeroCross=off
  mech limit pushes back?. : simulink/Logic and Bit Operations/Compare To Zero  relop=>  OutDataTypeStr=boolean  ZeroCross=off
  overextension angle : Constant  Value=mParams.joints.knee.MaxPitch
  overflexion angle : Constant  Value=mParams.joints.knee.MinPitch
  tau [Nm] : Outport  VectorParamsAs1DForOutWhenUnconnected=off
  wires:
  Gain5/1 -> Sum2/2
  Gain4/1 -> Gain2/1, Sum4/1
  const1/1 -> Sum4/2
  Sum4/1 -> Product2/3, mech limit pushes back?./1
  Gain1/1 -> Product2/2, below lower limit?/1
  mech limit pushes back?./1 -> Product2/4
  below lower limit?/1 -> Product2/1
  Product2/1 -> Gain5/1
  Product1/1 -> Gain6/1
  above upper limit?/1 -> Product1/1
  mech limit pushes back?/1 -> Product1/4
  Gain3/1 -> above upper limit?/1, Product1/2
  Sum3/1 -> mech limit pushes back?/1, Product1/3
  const/1 -> Sum3/2
  dq [rad/s]/1 -> Gain4/1
  overextension angle/1 -> Sum/2
  q [rad]/1 -> Sum/1, Limit Knee Range/1, Sum1/1
  Sum/1 -> Gain3/1
  Sum1/1 -> Gain1/1
  overflexion angle/1 -> Sum1/2
  Sum2/1 -> tau [Nm]/1
  Gain2/1 -> Sum3/1
  Gain6/1 -> Sum2/1
  Limit Knee Range/1 -> Logical Operator3/1
  Logical Operator3/1 -> Stop Simulation1/1

== system nms3D_2021/Body and Contact Model/L Leg/Rotation Sensor Knee ==
  note: Rotation Sensor in World Frame
  Coordinate Transformation Conversion2 : robotcorelib/Coordinate Transformation Conversion  InputRepresentation=Quaternion  InputEulerSequence=ZYX  ShowTrVecInputPort=on  OutputRepresentation=Rotation Matrix  OutputEulerSequence=XYZ  ShowTrVecOutputPort=on  SimulateUsing=Code generation
      settings: SourceProductBaseCode=NV,RO,RR,UV
  Frame Sensor : sm_lib/Frames and Transforms/Transform Sensor  MeasurementFrame=World  SenseAngle=off  SenseAxis=off  SenseAngle1=off  SenseAngle2=off  SenseAngle3=off  SenseQ=on  SenseR=off  SenseOmegaX=off  SenseOmegaY=off  SenseOmegaZ=off  SenseOmega1=off  SenseOmega2=off  SenseOmega3=off  SenseQDot=off  SenseRDot=off  SenseAlphaX=off  SenseAlphaY=off  SenseAlphaZ=off  SenseAlpha1=off  SenseAlpha2=off  SenseAlpha3=off  SenseQDDot=off  SenseRDDot=off  SenseX=off  SenseY=off  SenseZ=off  SenseRad=off  SenseAzim=off  SenseDist=off  SenseInc=off  SenseXDot=off  SenseYDot=off  SenseZDot=off  SenseRadDot=off  SenseAzimDot=off  SenseDistDot=off  SenseIncDot=off  SenseXDDot=off  SenseYDDot=off  SenseZDDot=off  SenseRadDDot=off  SenseAzimDDot=off  SenseDistDDot=off  SenseIncDDot=off
  PS-Simulink Converter12 : nesl_utility/PS-Simulink Converter  PhysicalDomain=network_engine_domain  SubClassName=ps_output  LeftPortType=input  RightPortType=output  PseudoPeriodic=off  Frequencies=[]  Unit=1  AffineConversion=off
      settings: SourceProductBaseCode=PW,SS
  World Frame : sm_lib/Frames and Transforms/World Frame
  frame : PMIOPort  Side=Left
  Rotation Matrix : Outport  VectorParamsAs1DForOutWhenUnconnected=off
  wires:
  PS-Simulink Converter12/1 -> Coordinate Transformation Conversion2/1
  Coordinate Transformation Conversion2/1 -> Rotation Matrix/1
  connections:
  Frame Sensor/RConn1 -- frame/RConn1
  World Frame/RConn1 -- Frame Sensor/LConn1
  PS-Simulink Converter12/LConn1 -- Frame Sensor/RConn2

== system nms3D_2021/Body and Contact Model/L Leg/Sensor Left Ankle ==
  note: Position and Velocity Sensor in World Frame
  Frame Sensor : sm_lib/Frames and Transforms/Transform Sensor  MeasurementFrame=Base  SenseAngle=off  SenseAxis=off  SenseAngle1=off  SenseAngle2=off  SenseAngle3=off  SenseQ=off  SenseR=off  SenseOmegaX=off  SenseOmegaY=off  SenseOmegaZ=off  SenseOmega1=off  SenseOmega2=off  SenseOmega3=off  SenseQDot=off  SenseRDot=off  SenseAlphaX=off  SenseAlphaY=off  SenseAlphaZ=off  SenseAlpha1=off  SenseAlpha2=off  SenseAlpha3=off  SenseQDDot=off  SenseRDDot=off  SenseX=on  SenseY=on  SenseZ=on  SenseRad=off  SenseAzim=off  SenseDist=off  SenseInc=off  SenseXDot=on  SenseYDot=on  SenseZDot=on  SenseRadDot=off  SenseAzimDot=off  SenseDistDot=off  SenseIncDot=off  SenseXDDot=off  SenseYDDot=off  SenseZDDot=off  SenseRadDDot=off  SenseAzimDDot=off  SenseDistDDot=off  SenseIncDDot=off
  Mux : Mux  Inputs=3
  Mux1 : Mux  Inputs=3
  PS-Simulink Converter1 : nesl_utility/PS-Simulink Converter  PhysicalDomain=network_engine_domain  SubClassName=ps_output  LeftPortType=input  RightPortType=output  PseudoPeriodic=off  Frequencies=[]  Unit=m  AffineConversion=off
      settings: SourceProductBaseCode=PW,SS
  PS-Simulink Converter12 : nesl_utility/PS-Simulink Converter  PhysicalDomain=network_engine_domain  SubClassName=ps_output  LeftPortType=input  RightPortType=output  PseudoPeriodic=off  Frequencies=[]  Unit=m  AffineConversion=off
      settings: SourceProductBaseCode=PW,SS
  PS-Simulink Converter2 : nesl_utility/PS-Simulink Converter  PhysicalDomain=network_engine_domain  SubClassName=ps_output  LeftPortType=input  RightPortType=output  PseudoPeriodic=off  Frequencies=[]  Unit=m  AffineConversion=off
      settings: SourceProductBaseCode=PW,SS
  PS-Simulink Converter3 : nesl_utility/PS-Simulink Converter  PhysicalDomain=network_engine_domain  SubClassName=ps_output  LeftPortType=input  RightPortType=output  PseudoPeriodic=off  Frequencies=[]  Unit=m/s  AffineConversion=off
      settings: SourceProductBaseCode=PW,SS
  PS-Simulink Converter4 : nesl_utility/PS-Simulink Converter  PhysicalDomain=network_engine_domain  SubClassName=ps_output  LeftPortType=input  RightPortType=output  PseudoPeriodic=off  Frequencies=[]  Unit=m/s  AffineConversion=off
      settings: SourceProductBaseCode=PW,SS
  PS-Simulink Converter5 : nesl_utility/PS-Simulink Converter  PhysicalDomain=network_engine_domain  SubClassName=ps_output  LeftPortType=input  RightPortType=output  PseudoPeriodic=off  Frequencies=[]  Unit=m/s  AffineConversion=off
      settings: SourceProductBaseCode=PW,SS
  World Frame : sm_lib/Frames and Transforms/World Frame
  Frame : PMIOPort  Side=Left
  Position [m] : Outport  VectorParamsAs1DForOutWhenUnconnected=off
  Velocity [m/s] : Outport  Port=2  VectorParamsAs1DForOutWhenUnconnected=off
  wires:
  PS-Simulink Converter12/1 -> Mux/1
  PS-Simulink Converter1/1 -> Mux/2
  PS-Simulink Converter2/1 -> Mux/3
  Mux/1 -> Position [m]/1
  PS-Simulink Converter5/1 -> Mux1/3
  PS-Simulink Converter4/1 -> Mux1/1
  Mux1/1 -> Velocity [m/s]/1
  PS-Simulink Converter3/1 -> Mux1/2
  connections:
  Frame Sensor/RConn1 -- Frame/RConn1
  PS-Simulink Converter12/LConn1 -- Frame Sensor/RConn2
  Frame Sensor/RConn3 -- PS-Simulink Converter1/LConn1
  Frame Sensor/RConn4 -- PS-Simulink Converter2/LConn1
  Frame Sensor/RConn7 -- PS-Simulink Converter5/LConn1
  Frame Sensor/RConn5 -- PS-Simulink Converter4/LConn1
  Frame Sensor/RConn6 -- PS-Simulink Converter3/LConn1
  World Frame/RConn1 -- Frame Sensor/LConn1

== system nms3D_2021/Body and Contact Model/L Leg/Shank ==
  Solid : sm_lib/Body Elements/Brick Solid  GraphicAmbientColor=[0.15 0.15 0.15 1.0]  BasedOnType=Density  BrickDimensions="[mParams.bodies.shank.d  mParams.bodies.shank.l mParams.bodies.shank.b]"  BrickDimensionUnits=m  CenterOfMass=mParams.bodies.shank.CG  CenterOfMassUnits=m  GraphicDiffuseColor=[1 0.5 0.5]  Density=2.7  DensityUnits=g/cm^3  DoExposeReferenceFrame=on  GraphicEmissiveColor=[0 0 0 1.0]  ExportEntireGeometry=off  SerializedFrames=<Frames><Frame><Id>Frame1</Id><Value><Name>F1</Name><Origin><Source>CenterOfMassFrame</Source><FeatureName></FeatureName></Origin><PrimaryAxis><DefinedDirection>+Z</DefinedDirection><Source>ReferenceFrame</Source><SourceDirection>+Z</SourceDirection><FeatureName></FeatureName></PrimaryAxis><SecondaryAxis><DefinedDirection>+X</DefinedDirection><Source>ReferenceFrame</Source><SourceDirection>+X</SourceDirection><FeatureName></FeatureName></SecondaryAxis></Value></Frame></Frames>  MarkerShape=Sphere  MarkerSize=10  GraphicType=FromGeometry  InertiaType=Custom  Mass=mParams.bodies.shank.m  MassUnits=kg  MomentsOfInertia=mParams.bodies.shank.In  MomentsOfInertiaUnits=kg*m^2  GraphicOpacity=1.0  ProductsOfInertia=[0 0 0]  ProductsOfInertiaUnits=kg*m^2  GraphicShininess=75  GraphicSpecularColor=[0.5 0.5 0.5 1.0]  GraphicVisPropType=SimpleVisualProperties
  Transform CS1 to MidSegment : sm_lib/Frames and Transforms/Rigid Transform  TranslationMethod=Cartesian  TranslationStandardOffset=0  TranslationLengthUnit=m  TranslationStandardAxis=+Y  TranslationCartesianOffset=[0 -mParams.bodies.shank.l/2 0]  TranslationROffset=0  TranslationROffsetUnits=m  TranslationZOffset=0  TranslationZOffsetUnits=m  TranslationThetaOffset=0  TranslationThetaOffsetUnits=deg  RotationMethod=None  RotationAngleUnits=deg  RotationStandardAxis=+X  RotationAngle=-90  RotationArbitraryAxis=[0 0 1]  FollAlignAxisA=+X  BaseAlignAxisA=+Y  FollAlignAxisB=+Y  BaseAlignAxisB=+Z  RotationSequenceAxes=FollowerAxes  RotationSequence=XYX  RotationSequenceAngles=[0 0 0]  RotationSequenceAnglesUnits=deg  RotationMatrix=[1 0 0; 0 1 0; 0 0 1]
  Transform MidSegment to CS2 : sm_lib/Frames and Transforms/Rigid Transform  TranslationMethod=Cartesian  TranslationStandardOffset=0  TranslationLengthUnit=m  TranslationStandardAxis=+Y  TranslationCartesianOffset=[ 0 -mParams.bodies.shank.l/2 0]  TranslationROffset=0  TranslationROffsetUnits=m  TranslationZOffset=0  TranslationZOffsetUnits=m  TranslationThetaOffset=0  TranslationThetaOffsetUnits=deg  RotationMethod=None  RotationAngleUnits=deg  RotationStandardAxis=+X  RotationAngle=90  RotationArbitraryAxis=[0 0 1]  FollAlignAxisA=+X  BaseAlignAxisA=+Y  FollAlignAxisB=+Y  BaseAlignAxisB=+Z  RotationSequenceAxes=FollowerAxes  RotationSequence=XYX  RotationSequenceAngles=[0 0 0]  RotationSequenceAnglesUnits=deg  RotationMatrix=[1 0 0; 0 1 0; 0 0 1]
  CS1 : PMIOPort  Side=Left
  CS2 : PMIOPort  Port=2  Side=Right
  connections:
  Transform MidSegment to CS2/RConn1 -- CS2/RConn1
  Transform CS1 to MidSegment/LConn1 -- CS1/RConn1
  Solid/RConn1 -- Transform CS1 to MidSegment/RConn1 -- Transform MidSegment to CS2/LConn1

== system nms3D_2021/Body and Contact Model/L Leg/Thigh ==
  Solid : sm_lib/Body Elements/Brick Solid  Commented=on  GraphicAmbientColor=[0.15 0.15 0.15 1.0]  BasedOnType=Density  BrickDimensions="[mParams.bodies.thigh.d  mParams.bodies.thigh.l*(1-mParams.bodies.thigh.ThPos)   mParams.bodies.thigh.b]"  BrickDimensionUnits=m  CenterOfMass=-mParams.bodies.thigh.CG*(1-mParams.bodies.thigh.ThPos)  CenterOfMassUnits=m  GraphicDiffuseColor=[1 0.5 0.5]  Density=2.7  DensityUnits=g/cm^3  DoExposeReferenceFrame=on  GraphicEmissiveColor=[0 0 0 1.0]  ExportEntireGeometry=off  SerializedFrames=<Frames/>  MarkerShape=Sphere  MarkerSize=10  GraphicType=FromGeometry  InertiaType=Custom  Mass=mParams.bodies.thigh.m*(1-mParams.bodies.thigh.ThPos)  MassUnits=kg  MomentsOfInertia=mParams.bodies.thigh.In*[(1-mParams.bodies.thigh.ThPos); (1-mParams.bodies.thigh.ThPos)^3; (1-mParams.bodies.thigh.ThPos)^3]  MomentsOfInertiaUnits=kg*m^2  GraphicOpacity=1.0  ProductsOfInertia=[0 0 0]  ProductsOfInertiaUnits=kg*m^2  GraphicShininess=75  GraphicSpecularColor=[0.5 0.5 0.5 1.0]  GraphicVisPropType=SimpleVisualProperties
  Solid1 : sm_lib/Body Elements/Brick Solid  GraphicAmbientColor=[0.15 0.15 0.15 1.0]  BasedOnType=Density  BrickDimensions=[mParams.bodies.thigh.d mParams.bodies.thigh.l mParams.bodies.thigh.b]  BrickDimensionUnits=m  CenterOfMass=mParams.bodies.thigh.CG  CenterOfMassUnits=m  GraphicDiffuseColor=[1 0.5 0.5]  Density=2.7  DensityUnits=g/cm^3  DoExposeReferenceFrame=on  GraphicEmissiveColor=[0 0 0 1.0]  ExportEntireGeometry=off  SerializedFrames=<Frames><Frame><Id>Frame1</Id><Value><Name>F1</Name><Origin><Source>CenterOfMassFrame</Source><FeatureName></FeatureName></Origin><PrimaryAxis><DefinedDirection>+Z</DefinedDirection><Source>ReferenceFrame</Source><SourceDirection>+Z</SourceDirection><FeatureName></FeatureName></PrimaryAxis><SecondaryAxis><DefinedDirection>+X</DefinedDirection><Source>ReferenceFrame</Source><SourceDirection>+X</SourceDirection><FeatureName></FeatureName></SecondaryAxis></Value></Frame></Frames>  MarkerShape=Sphere  MarkerSize=10  GraphicType=FromGeometry  InertiaType=Custom  Mass=mParams.bodies.thigh.m  MassUnits=kg  MomentsOfInertia=mParams.bodies.thigh.In  MomentsOfInertiaUnits=kg*m^2  GraphicOpacity=1.0  ProductsOfInertia=[0 0 0]  ProductsOfInertiaUnits=kg*m^2  GraphicShininess=75  GraphicSpecularColor=[0.5 0.5 0.5 1.0]  GraphicVisPropType=SimpleVisualProperties
  Transform CG to MidSegment : sm_lib/Frames and Transforms/Rigid Transform  TranslationMethod=Cartesian  TranslationStandardOffset=0  TranslationLengthUnit=m  TranslationStandardAxis=+Y  TranslationCartesianOffset=[0 -mParams.bodies.thigh.l/2 0]  TranslationROffset=0  TranslationROffsetUnits=m  TranslationZOffset=0  TranslationZOffsetUnits=m  TranslationThetaOffset=0  TranslationThetaOffsetUnits=deg  RotationMethod=None  RotationAngleUnits=deg  RotationStandardAxis=+X  RotationAngle=90  RotationArbitraryAxis=[0 0 1]  FollAlignAxisA=+X  BaseAlignAxisA=+Y  FollAlignAxisB=+Y  BaseAlignAxisB=+Z  RotationSequenceAxes=FollowerAxes  RotationSequence=XYX  RotationSequenceAngles=[0 0 0]  RotationSequenceAnglesUnits=deg  RotationMatrix=[1 0 0; 0 1 0; 0 0 1]
  Transform CS1 to MidSegment : sm_lib/Frames and Transforms/Rigid Transform  TranslationMethod=Cartesian  TranslationStandardOffset=0  TranslationLengthUnit=m  TranslationStandardAxis=+Y  TranslationCartesianOffset=[0 -mParams.bodies.thigh.l/2 0]  TranslationROffset=0  TranslationROffsetUnits=m  TranslationZOffset=0  TranslationZOffsetUnits=m  TranslationThetaOffset=0  TranslationThetaOffsetUnits=deg  RotationMethod=None  RotationAngleUnits=deg  RotationStandardAxis=+X  RotationAngle=-90  RotationArbitraryAxis=[0 0 1]  FollAlignAxisA=+X  BaseAlignAxisA=+Y  FollAlignAxisB=+Y  BaseAlignAxisB=+Z  RotationSequenceAxes=FollowerAxes  RotationSequence=XYX  RotationSequenceAngles=[0 0 0]  RotationSequenceAnglesUnits=deg  RotationMatrix=[1 0 0; 0 1 0; 0 0 1]
  CS1 : PMIOPort  Side=Left
  CS2 : PMIOPort  Port=2  Side=Right
  connections:
  Transform CG to MidSegment/LConn1 -- Solid1/RConn1 -- Transform CS1 to MidSegment/RConn1
  Transform CS1 to MidSegment/LConn1 -- CS1/RConn1
  Transform CG to MidSegment/RConn1 -- CS2/RConn1
